simulink model "reference"  (Simulink 6.2)
settings: Solver=FixedStepDiscrete  StartTime=0.0  StopTime=st  FixedStep=Ts  RelTol=1e-3
values from neighbouring files (symbols this model uses):
  a0 = alpha(1)    [Ex8_1Launch.m]
  a1 = alpha(2)    [Ex8_1Launch.m]
  a2 = alpha(3)    [Ex8_1Launch.m]
  a3 = alpha(4)    [Ex8_1Launch.m]
  a4 = alpha(5)    [Ex8_1Launch.m]
  a5 = alpha(6)    [Ex8_1Launch.m]
  a6 = alpha(7)    [Ex8_1Launch.m]
  Fin = nper*Fs/N    (= 0.271240234375)    [Ex8_1Launch.m]
  flag = -1    [Ex8_1Launch.m]
  i1 = ic(1)*D    [Ex8_1Launch.m]
  i2 = ic(2)*D    [Ex8_1Launch.m]
  i3 = ic(3)*D    [Ex8_1Launch.m]
  i4 = ic(4)*D    [Ex8_1Launch.m]
  i5 = ic(5)*D    [Ex8_1Launch.m]
  i6 = ic(6)*D    [Ex8_1Launch.m]
  i7 = ic(7)*D    [Ex8_1Launch.m]
  i8 = ic(8)*D    [Ex8_1Launch.m]
  Ts = 1/Fs    (= 1)    [Ex8_1Launch.m]
undefined symbols (not defined in the file or in its folder): conversion
settings Model: Creator=francomaloberti  LastModifiedBy=francomaloberti  ExtModeAutoUpdateStatusClock=off
settings SolverCC: AutoInsertRateTranBlk=on
settings OptimizationCC: InlineInvariantSignals=on
settings DebuggingCC: SolverPrmCheckMsg=warning

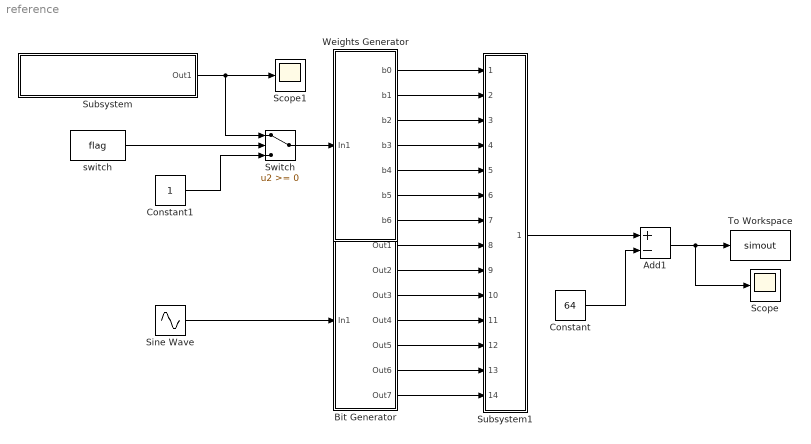
== system reference ==
  Add1 : Sum  Inputs=+-  OutDataTypeMode=double  OutScaling=2^-10
  Bit Generator : Subsystem
  Constant : Constant  Value=64
  Constant1 : Constant
  Scope : Scope
      settings: YMin=-70  YMax=70
  Scope1 : Scope
      settings: YMin=-70  YMax=70  SaveName=ScopeData2
  Sine Wave : Sin  Amplitude=63  Bias=64  Frequency=Fin  Phase=pi/7  SampleTime=Ts
  Subsystem : Subsystem
      mask Display: color('red');disp('RANDOM NOISE GENERATOR')
  Subsystem1 : Subsystem
  Switch : Switch
  To Workspace : ToWorkspace  VariableName=simout  SampleTime=Ts  SaveFormat=Array
  Weights Generator : Subsystem
  switch : Constant  Value=flag
  wires:
  Weights Generator/1(b0) -> Subsystem1/1(In1)
  Weights Generator/2(b1) -> Subsystem1/2(In2)
  Sine Wave/1 -> Bit Generator/1(In1)
  Subsystem1/1(Out1) -> Add1/1
  Constant/1 -> Add1/2
  Add1/1 -> Scope/1, To Workspace/1
  Switch/1 -> Weights Generator/1(In1)
  Subsystem/1(Out1) -> Switch/1, Scope1/1
  Constant1/1 -> Switch/3
  switch/1 -> Switch/2
  Weights Generator/3(b2) -> Subsystem1/3(In3)
  Weights Generator/4(b3) -> Subsystem1/4(In4)
  Weights Generator/5(b4) -> Subsystem1/5(In5)
  Weights Generator/6(b5) -> Subsystem1/6(In6)
  Weights Generator/7(b6) -> Subsystem1/7(In7)
  Bit Generator/1(Out1) -> Subsystem1/8(In8)
  Bit Generator/2(Out2) -> Subsystem1/9(In9)
  Bit Generator/3(Out3) -> Subsystem1/10(In10)
  Bit Generator/4(Out4) -> Subsystem1/11(In11)
  Bit Generator/5(Out5) -> Subsystem1/12(In12)
  Bit Generator/6(Out6) -> Subsystem1/13(In13)
  Bit Generator/7(Out7) -> Subsystem1/14(In14)

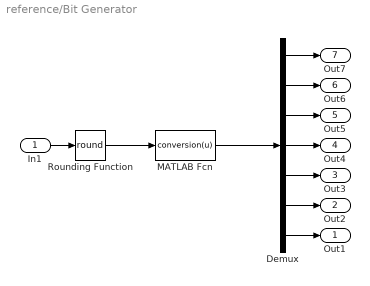
== system reference/Bit Generator ==
  In1 : Inport  Port=1  LatchInput=off
  Demux : Demux  Outputs=7
  MATLAB Fcn : MATLABFcn  MATLABFcn=conversion(u)  OutputDimensions=7  OutputSignalType=real  Output1D=off
  Rounding Function : Rounding  Operator=round
  Out1 : Outport
  Out2 : Outport  Port=2
  Out3 : Outport  Port=3
  Out4 : Outport  Port=4
  Out5 : Outport  Port=5
  Out6 : Outport  Port=6
  Out7 : Outport  Port=7
  wires:
  MATLAB Fcn/1 -> Demux/1
  Rounding Function/1 -> MATLAB Fcn/1
  In1/1 -> Rounding Function/1
  Demux/7 -> Out1/1
  Demux/6 -> Out2/1
  Demux/5 -> Out3/1
  Demux/4 -> Out4/1
  Demux/3 -> Out5/1
  Demux/2 -> Out6/1
  Demux/1 -> Out7/1

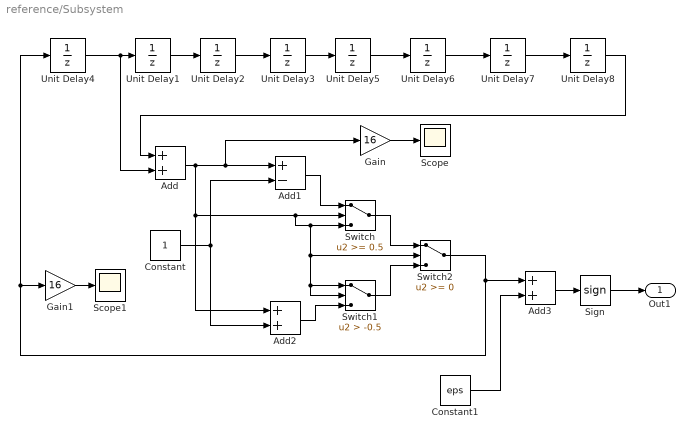
== system reference/Subsystem ==
  Add : Sum  OutDataTypeMode=double  OutScaling=2^-10
  Add1 : Sum  Inputs=+-  OutDataTypeMode=double  OutScaling=2^-10
  Add2 : Sum  OutDataTypeMode=double  OutScaling=2^-10
  Add3 : Sum  OutDataTypeMode=double  OutScaling=2^-10
  Constant : Constant
  Constant1 : Constant  Value=eps
  Gain : Gain  Gain=16
  Gain1 : Gain  Gain=16
  Scope : Scope
  Scope1 : Scope
      settings: SaveName=ScopeData3
  Sign : Signum
  Switch : Switch  Threshold=0.5
  Switch1 : Switch  Criteria=u2 > Threshold  Threshold=-0.5
  Switch2 : Switch
  Unit Delay1 : UnitDelay  X0=i2
  Unit Delay2 : UnitDelay  X0=i3
  Unit Delay3 : UnitDelay  X0=i4
  Unit Delay4 : UnitDelay  X0=i1
  Unit Delay5 : UnitDelay  X0=i5
  Unit Delay6 : UnitDelay  X0=i6
  Unit Delay7 : UnitDelay  X0=i7
  Unit Delay8 : UnitDelay  X0=i8
  Out1 : Outport
  wires:
  Unit Delay4/1 -> Unit Delay1/1, Add/2
  Unit Delay1/1 -> Unit Delay2/1
  Unit Delay2/1 -> Unit Delay3/1
  Unit Delay7/1 -> Unit Delay8/1
  Unit Delay8/1 -> Add/1
  Unit Delay3/1 -> Unit Delay5/1
  Unit Delay5/1 -> Unit Delay6/1
  Unit Delay6/1 -> Unit Delay7/1
  Add/1 -> Switch/2, Switch2/2, Switch1/2, Switch1/1, Switch/3, Add2/1, Add1/1, Gain/1
  Constant/1 -> Add1/2, Add2/2
  Add2/1 -> Switch1/3
  Switch/1 -> Switch2/1
  Switch1/1 -> Switch2/3
  Switch2/1 -> Add3/1, Unit Delay4/1, Gain1/1
  Add1/1 -> Switch/1
  Sign/1 -> Out1/1
  Add3/1 -> Sign/1
  Constant1/1 -> Add3/2
  Gain/1 -> Scope/1
  Gain1/1 -> Scope1/1

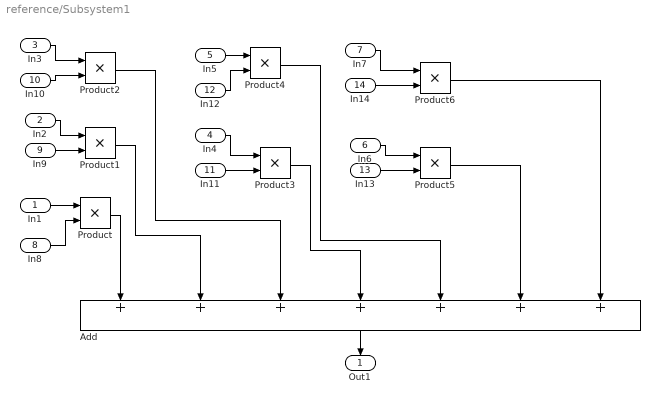
== system reference/Subsystem1 ==
  In1 : Inport  Port=1  LatchInput=off
  In2 : Inport  Port=2  LatchInput=off
  In3 : Inport  Port=3  LatchInput=off
  In4 : Inport  Port=4  LatchInput=off
  In5 : Inport  Port=5  LatchInput=off
  In6 : Inport  Port=6  LatchInput=off
  In7 : Inport  Port=7  LatchInput=off
  In8 : Inport  Port=8  LatchInput=off
  In9 : Inport  Port=9  LatchInput=off
  In10 : Inport  Port=10  LatchInput=off
  In11 : Inport  Port=11  LatchInput=off
  In12 : Inport  Port=12  LatchInput=off
  In13 : Inport  Port=13  LatchInput=off
  In14 : Inport  Port=14  LatchInput=off
  Add : Sum  Orientation=down  Inputs=+++++++  OutDataTypeMode=double  OutScaling=2^-10  SampleTime=Ts  InputSameDT=on
  Product{,1..6} (7 alike) : Product  RndMeth=Zero
  Out1 : Outport  Orientation=down
  wires:
  Product1/1 -> Add/2
  Product2/1 -> Add/3
  Product3/1 -> Add/4
  Product4/1 -> Add/5
  Product5/1 -> Add/6
  Product6/1 -> Add/7
  Product/1 -> Add/1
  In1/1 -> Product/1
  In2/1 -> Product1/1
  In3/1 -> Product2/1
  In4/1 -> Product3/1
  In5/1 -> Product4/1
  In6/1 -> Product5/1
  In7/1 -> Product6/1
  In8/1 -> Product/2
  In9/1 -> Product1/2
  In10/1 -> Product2/2
  In11/1 -> Product3/2
  In13/1 -> Product5/2
  In14/1 -> Product6/2
  Add/1 -> Out1/1
  In12/1 -> Product4/2

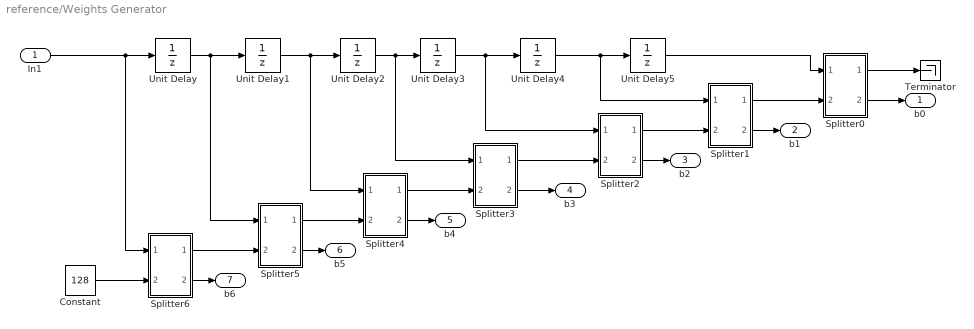
== system reference/Weights Generator ==
  In1 : Inport  Port=1  LatchInput=off
  Constant : Constant  Value=128
  Splitter0 : Subsystem
  Splitter1 : Subsystem
  Splitter2 : Subsystem
  Splitter3 : Subsystem
  Splitter4 : Subsystem
  Splitter5 : Subsystem
  "Splitter6 " : Subsystem
  Terminator : Terminator
  Unit Delay{,1..5} (6 alike) : UnitDelay  SampleTime=Ts
  b0 : Outport  DataType=double
  b1 : Outport  Port=2  SampleTime=Ts  DataType=double
  b2 : Outport  Port=3  DataType=double
  b3 : Outport  Port=4  DataType=double
  b4 : Outport  Port=5
  b5 : Outport  Port=6
  b6 : Outport  Port=7  DataType=double
  wires:
  In1/1 -> Unit Delay/1, "Splitter6 "/1(In1)
  Splitter0/1(Out1) -> Terminator/1
  "Splitter6 "/2(Out2) -> b6/1
  Splitter4/2(Out2) -> b4/1
  Splitter3/2(Out2) -> b3/1
  Splitter2/2(Out2) -> b2/1
  Splitter1/2(Out2) -> b1/1
  Splitter0/2(Out2) -> b0/1
  Unit Delay/1 -> Unit Delay1/1, Splitter5/1(In1)
  Unit Delay1/1 -> Unit Delay2/1, Splitter4/1(In1)
  Unit Delay2/1 -> Unit Delay3/1, Splitter3/1(In1)
  Unit Delay3/1 -> Unit Delay4/1, Splitter2/1(In1)
  Unit Delay4/1 -> Unit Delay5/1, Splitter1/1(In1)
  Constant/1 -> "Splitter6 "/2(In2)
  "Splitter6 "/1(Out1) -> Splitter5/2(In2)
  Splitter5/2(Out2) -> b5/1
  Splitter5/1(Out1) -> Splitter4/2(In2)
  Splitter4/1(Out1) -> Splitter3/2(In2)
  Splitter3/1(Out1) -> Splitter2/2(In2)
  Splitter2/1(Out1) -> Splitter1/2(In2)
  Unit Delay5/1 -> Splitter0/1(In1)
  Splitter1/1(Out1) -> Splitter0/2(In2)

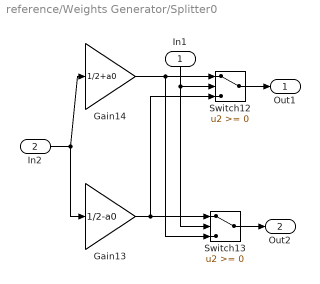
== system reference/Weights Generator/Splitter0 ==
  In1 : Inport  Orientation=down  Port=1  LatchInput=off
  In2 : Inport  Port=2  LatchInput=off
  Gain13 : Gain  Gain=1/2-a0
  Gain14 : Gain  Gain=1/2+a0
  Switch12 : Switch
  Switch13 : Switch
  Out1 : Outport
  Out2 : Outport  Port=2
  wires:
  In2/1 -> Gain13/1, Gain14/1
  Gain14/1 -> Switch12/1, Switch13/3
  Gain13/1 -> Switch13/1, Switch12/3
  In1/1 -> Switch12/2, Switch13/2
  Switch12/1 -> Out1/1
  Switch13/1 -> Out2/1

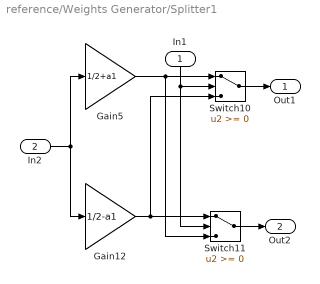
== system reference/Weights Generator/Splitter1 ==
  In1 : Inport  Orientation=down  Port=1  LatchInput=off
  In2 : Inport  Port=2  LatchInput=off
  Gain12 : Gain  Gain=1/2-a1
  Gain5 : Gain  Gain=1/2+a1
  Switch10 : Switch
  Switch11 : Switch
  Out1 : Outport
  Out2 : Outport  Port=2
  wires:
  In2/1 -> Gain12/1, Gain5/1
  Gain5/1 -> Switch10/1, Switch11/3
  Gain12/1 -> Switch11/1, Switch10/3
  In1/1 -> Switch11/2, Switch10/2
  Switch10/1 -> Out1/1
  Switch11/1 -> Out2/1

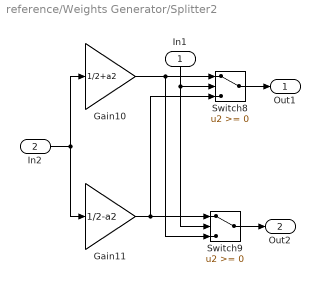
== system reference/Weights Generator/Splitter2 ==
  In1 : Inport  Orientation=down  Port=1  LatchInput=off
  In2 : Inport  Port=2  LatchInput=off
  Gain10 : Gain  Gain=1/2+a2
  Gain11 : Gain  Gain=1/2-a2
  Switch8 : Switch
  Switch9 : Switch
  Out1 : Outport
  Out2 : Outport  Port=2
  wires:
  In2/1 -> Gain11/1, Gain10/1
  Gain10/1 -> Switch8/1, Switch9/3
  Gain11/1 -> Switch9/1, Switch8/3
  In1/1 -> Switch9/2, Switch8/2
  Switch8/1 -> Out1/1
  Switch9/1 -> Out2/1

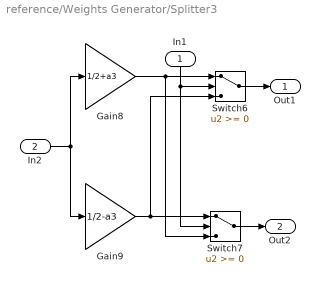
== system reference/Weights Generator/Splitter3 ==
  In1 : Inport  Orientation=down  Port=1  LatchInput=off
  In2 : Inport  Port=2  LatchInput=off
  Gain8 : Gain  Gain=1/2+a3
  Gain9 : Gain  Gain=1/2-a3
  Switch6 : Switch
  Switch7 : Switch
  Out1 : Outport
  Out2 : Outport  Port=2
  wires:
  In2/1 -> Gain9/1, Gain8/1
  Gain8/1 -> Switch6/1, Switch7/3
  Gain9/1 -> Switch7/1, Switch6/3
  In1/1 -> Switch7/2, Switch6/2
  Switch6/1 -> Out1/1
  Switch7/1 -> Out2/1

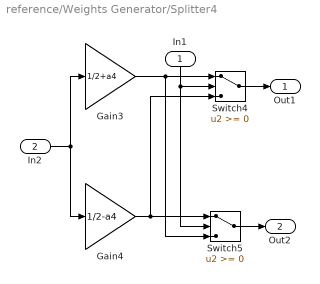
== system reference/Weights Generator/Splitter4 ==
  In1 : Inport  Orientation=down  Port=1  LatchInput=off
  In2 : Inport  Port=2  LatchInput=off
  Gain3 : Gain  Gain=1/2+a4
  Gain4 : Gain  Gain=1/2-a4
  Switch4 : Switch
  Switch5 : Switch
  Out1 : Outport
  Out2 : Outport  Port=2
  wires:
  In2/1 -> Gain4/1, Gain3/1
  Gain3/1 -> Switch4/1, Switch5/3
  Gain4/1 -> Switch5/1, Switch4/3
  In1/1 -> Switch5/2, Switch4/2
  Switch4/1 -> Out1/1
  Switch5/1 -> Out2/1

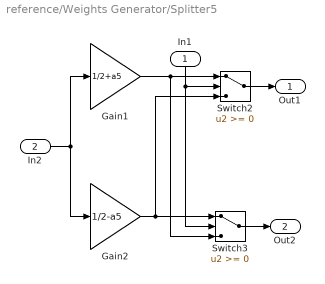
== system reference/Weights Generator/Splitter5 ==
  In1 : Inport  Orientation=down  Port=1  LatchInput=off
  In2 : Inport  Port=2  LatchInput=off
  Gain1 : Gain  Gain=1/2+a5
  Gain2 : Gain  Gain=1/2-a5
  Switch2 : Switch
  Switch3 : Switch
  Out1 : Outport
  Out2 : Outport  Port=2
  wires:
  In2/1 -> Gain2/1, Gain1/1
  Gain1/1 -> Switch2/1, Switch3/3
  Gain2/1 -> Switch3/1, Switch2/3
  In1/1 -> Switch3/2, Switch2/2
  Switch2/1 -> Out1/1
  Switch3/1 -> Out2/1

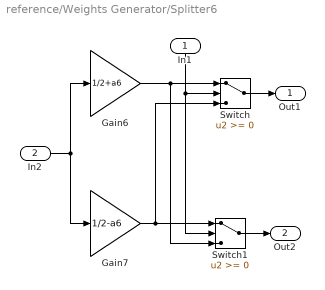
== system reference/Weights Generator/Splitter6  ==
  In1 : Inport  Orientation=down  Port=1  LatchInput=off
  In2 : Inport  Port=2  LatchInput=off
  Gain6 : Gain  Gain=1/2+a6
  Gain7 : Gain  Gain=1/2-a6
  Switch : Switch
  Switch1 : Switch
  Out1 : Outport
  Out2 : Outport  Port=2
  wires:
  In2/1 -> Gain7/1, Gain6/1
  Gain6/1 -> Switch/1, Switch1/3
  Gain7/1 -> Switch1/1, Switch/3
  In1/1 -> Switch/2, Switch1/2
  Switch/1 -> Out1/1
  Switch1/1 -> Out2/1
